simulink model "reg_lqr3"  (R2016a)
settings: Solver=VariableStepAuto  StartTime=0.0  StopTime=10.0  RelTol=1e-3
values from neighbouring files (symbols this model uses):
  Al = [0  1     0 0 ... (first row only)    [cel.m]    (also in req_lqr.m; zobserwatorem.m)
  Bl = [0; Km/T; 0; K*Km*omega^2/T]    [cel.m]    (also in req_lqr.m; zobserwatorem.m)
  Klqr = lqr(Al,Bl,Q,R)    [cel.m]    (also in req_lqr.m)
  X0 = [0 0 0 0]    [cel.m]    (also in celPID.m = [0 0]; min_PID.m = [0 0]; pod_discPID.m = [0 0]; por_model_obiekt_osX.m = [0 0])
settings Model: Creator=Maciek  LastModifiedBy=Maciek

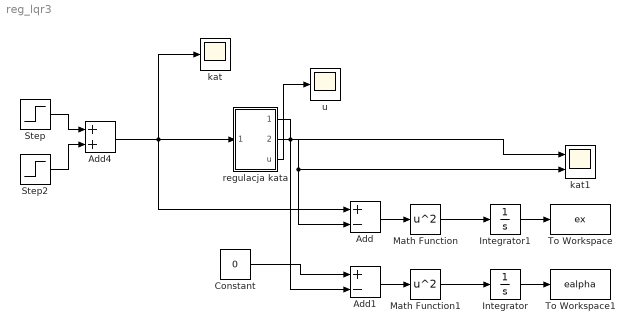
== system reg_lqr3 ==
  Add : Sum  Inputs=+-
  Add1 : Sum  Inputs=+-
  Add4 : Sum
  Constant : Constant  Value=0
  Integrator : Integrator
  Integrator1 : Integrator
  Math Function : Math  Operator=square  SaturateOnIntegerOverflow=on
  Math Function1 : Math  Operator=square  SaturateOnIntegerOverflow=on
  Step : Step  After=0.2  SampleTime=0
  Step2 : Step  Time=40  After=-0.7  SampleTime=0
  To Workspace : ToWorkspace  VariableName=ex  SampleTime=-1
      settings: MaxDataPoints=1
  To Workspace1 : ToWorkspace  VariableName=ealpha  SampleTime=-1
      settings: MaxDataPoints=1
  kat : Scope
  kat1 : Scope  NumInputPorts=2
  regulacja kata : Subsystem
  u : Scope
  wires:
  Step/1 -> Add4/1
  Step2/1 -> Add4/2
  regulacja kata/3(u) -> u/1
  regulacja kata/1(alpha) -> Add1/2, kat1/1
  regulacja kata/2(pol) -> Add/2, kat1/2
  Add4/1 -> kat/1, Add/1, regulacja kata/1(zad)
  Add/1 -> Math Function/1
  Add1/1 -> Math Function1/1
  Math Function1/1 -> Integrator/1
  Math Function/1 -> Integrator1/1
  Integrator1/1 -> To Workspace/1
  Integrator/1 -> To Workspace1/1
  Constant/1 -> Add1/1

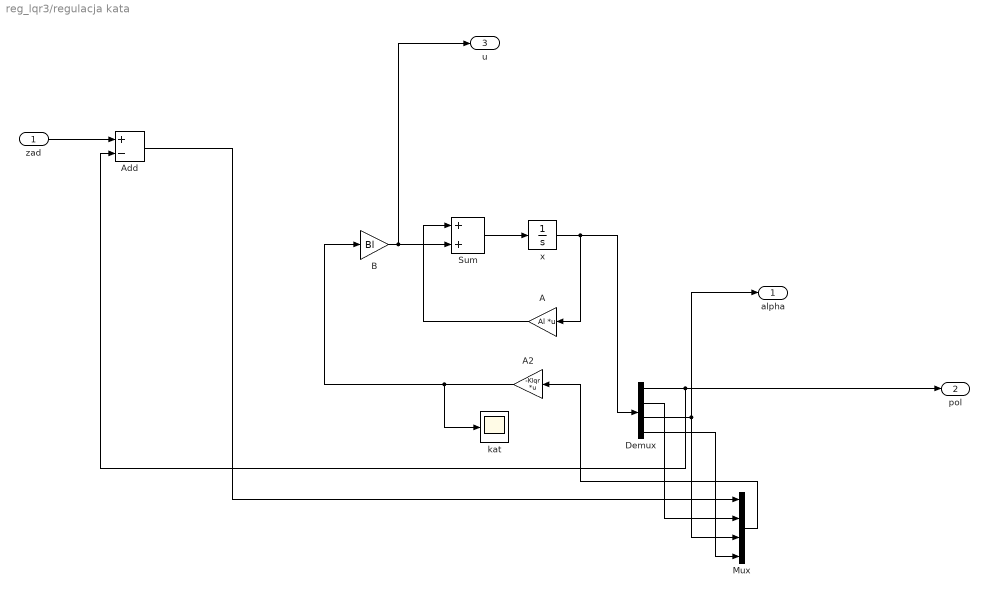
== system reg_lqr3/regulacja kata ==
  zad : Inport
  A : Gain  Gain=Al  Multiplication=Matrix(K*u) (u vector)
  A2 : Gain  Gain=-Klqr  Multiplication=Matrix(K*u) (u vector)
  Add : Sum  Inputs=+-
  B : Gain  Gain=Bl
  Demux : Demux
  Mux : Mux
  Sum : Sum
  kat : Scope
  x : Integrator  InitialCondition=X0
  alpha : Outport
  pol : Outport  Port=2
  u : Outport  Port=3
  wires:
  zad/1 -> Add/1
  Sum/1 -> x/1
  x/1 -> A/1, Demux/1
  B/1 -> u/1, Sum/2
  A2/1 -> kat/1, B/1
  Demux/1 -> pol/1, Add/2
  Demux/3 -> Mux/3, alpha/1
  Add/1 -> Mux/1
  Demux/2 -> Mux/2
  Demux/4 -> Mux/4
  Mux/1 -> A2/1
  A/1 -> Sum/1
